simulink model "Chap7_OFDM"  (R2016a)
settings: Solver=VariableStepDiscrete  StartTime=0.0  StopTime=SimTime  RelTol=1e-3
InitFcn:
  | DopplerShift = 10; % 最大多普勒频移，单位Hz
  | % LTE EPA信道模型
  | Tau = ([0 30 70 90 110 190 410]) * 1e-9; % 每径的延迟，单位s
  | Pdb = [0 -1.0 -2.0 -3.0 -8.0 -17.2 -20.8]; % 每径的功率衰减
  | SNR = 10; % 信噪比
  | SimTime = 5; % 仿真时间
undefined symbols (not defined in the file or in its folder): clock
libraries: dspmtrx3 x12, dspxfrm3 x4, commchan3 x3, commdigbbndam3 x3, commrandsrc2 x2, commsink2 x1
settings Model: Creator=Administrator  LastModifiedBy=Administrator
settings DataIOCC: LimitDataPoints=on  SaveFormat=Array
settings DebuggingCC: SignalRangeChecking=warning  ParameterOverflowMsg=warning  ParameterPrecisionLossMsg=none  ParameterTunabilityLossMsg=none
settings HardwareCC: ProdBitPerPointer=32  ProdLargestAtomicFloat=None  ProdIntDivRoundTo=Undefined  ProdEndianess=Unspecified  ProdWordSize=32  ProdHWDeviceType=ASIC/FPGA->ASIC/FPGA  TargetHWDeviceType=Generic->Custom  ProdEqTarget=off
settings ModelReferenceCC: PropagateSignalLabelsOutOfModel=off
settings ConfigComp: CovModelRefEnable=Off

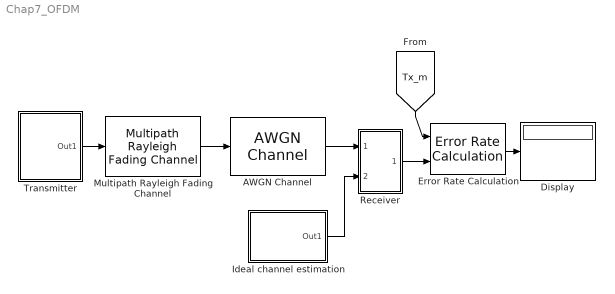
== system Chap7_OFDM ==
  AWGN Channel : commchan3/AWGN Channel  InputProcessing=Columns as channels (frame based)  seed=67  noiseMode=Variance from mask  EbNodB=10  EsNodB=10  SNRdB=10  bitsPerSym=1  Ps=1  Tsym=1  variance=1200/2048/(10^(SNR/10))
  Display : Display
  Error Rate Calculation : commsink2/Error Rate Calculation  N=0  st_delay=0  cp_mode=Entire frame  subframe=[]  PMode=Port  WsName=ErrorVec  RsMode2=off  stop=off  numErr=100  maxBits=1e6
  Ideal channel estimation : Subsystem
  Multipath Rayleigh Fading Channel : commchan3/Multipath Rayleigh Fading Channel  maxDopplerShift=10  spectrumType=Jakes  sigmaGaussian=1/sqrt(2)  coeffRounded=[1 -1.72 0.785]  freqMinMaxRJakes=[0 1]  freqMinMaxAJakes=[0 1]  sigmaGaussian1=1/sqrt(2)  sigmaGaussian2=1/sqrt(2)  centerFreqGaussian1=0.0  centerFreqGaussian2=0.0  gainGaussian1=0.5  gainGaussian2=0.5  coeffBell=9  dopplerSpectrum=doppler.jakes  pathDelays=Tau  avgPathGaindB=Pdb  normalizePathGains=on  seed=73  enableProbe=0  openVisAtStart=off  outPathGains=off  outDelay=off
  Receiver : Subsystem
  Transmitter : Subsystem
  wires:
  Multipath Rayleigh Fading Channel/1 -> AWGN Channel/1
  Error Rate Calculation/1 -> Display/1
  Transmitter/1(Out1) -> Multipath Rayleigh Fading Channel/1
  AWGN Channel/1 -> Receiver/1(In1)
  Ideal channel estimation/1(Out1) -> Receiver/2(In2)
  Receiver/1(Out1) -> Error Rate Calculation/2
  [Tx_m] -> Error Rate Calculation/1

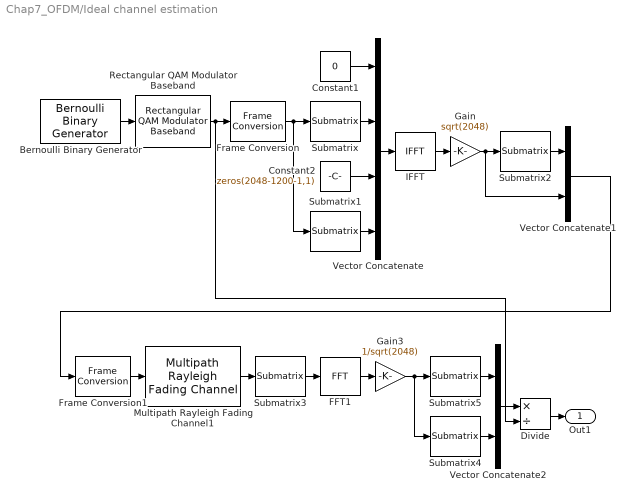
== system Chap7_OFDM/Ideal channel estimation ==
  Bernoulli Binary Generator : commrandsrc2/Bernoulli Binary Generator  P=0  seed=round(100*sum(clock))  Ts=0.5e-3/(1200*4)  frameBased=on  sampPerFrame=1200*4  orient=off  outDataType=double
  Constant1 : Constant  Value=0
  Constant2 : Constant  Value=zeros(2048-1200-1,1)
  Divide : Product  Inputs=*/
  FFT1 : dspxfrm3/FFT  FFTImplementation=Auto  CompMethod=Table lookup  TableOpt=NEW  TableOptActive=Speed  BitRevOrder=off  Normalize=off  InheritFFTLength=on  FFTLength=64  WrapInput=on  roundingMode=Floor  overflowMode=off  firstCoeffDataTypeStr=Inherit: Same word length as input  firstCoeffLastDataTypeStr=Inherit: Same word length as input  outputMin=[]  outputMax=[]
  Frame Conversion : FrameConversion  InheritSamplingMode=off  OutFrame=Sample-based
  Frame Conversion1 : FrameConversion  InheritSamplingMode=off
  Gain : Gain  Gain=sqrt(2048)
  Gain3 : Gain  Gain=1/sqrt(2048)
  IFFT : dspxfrm3/IFFT  FFTImplementation=Auto  CompMethod=Table lookup  TableOpt=NEW  TableOptActive=Speed  BitRevOrder=off  cs_in=off  Normalize=on  InheritFFTLength=on  FFTLength=64  WrapInput=on  mode=Complex  outSamplingMode=Sample based  roundingMode=Floor  overflowMode=off  firstCoeffDataTypeStr=Inherit: Same word length as input  firstCoeffLastDataTypeStr=Inherit: Same word length as input  outputMin=[]  outputMax=[]
  Multipath Rayleigh Fading Channel1 : commchan3/Multipath Rayleigh Fading Channel  maxDopplerShift=DopplerShift  spectrumType=Jakes  sigmaGaussian=1/sqrt(2)  coeffRounded=[1 -1.72 0.785]  freqMinMaxRJakes=[0 1]  freqMinMaxAJakes=[0 1]  sigmaGaussian1=1/sqrt(2)  sigmaGaussian2=1/sqrt(2)  centerFreqGaussian1=0.0  centerFreqGaussian2=0.0  gainGaussian1=0.5  gainGaussian2=0.5  coeffBell=9  dopplerSpectrum=doppler.jakes  pathDelays=Tau  avgPathGaindB=Pdb  normalizePathGains=on  seed=73  enableProbe=0  openVisAtStart=off  outPathGains=off  outDelay=off
  Rectangular QAM Modulator Baseband : commdigbbndam3/Rectangular QAM Modulator Baseband  M=16  InType=Bit  Enc=Gray  Mapping=[0:15]  PowType=Average Power  MinDist=2  AvgPow=1  PeakPow=1  Ph=0  outDtype=double  outWordLen=16  outUDDataType=sfix(16)  outFracLenMode=Best precision  outFracLen=15  outDataTypeStr=double  outLastDataTypeStr=double
  Submatrix : dspmtrx3/Submatrix  RowSpan=Range of rows  RowStartMode=Index  RowStartIndex=601  RowEndMode=Last  RowEndIndex=600  ColSpan=All columns  ColStartMode=First  ColStartIndex=1  ColEndMode=Last  ColEndIndex=1
  Submatrix1 : dspmtrx3/Submatrix  RowSpan=Range of rows  RowStartMode=First  RowStartIndex=1  RowEndMode=Index  RowEndIndex=600  ColSpan=All columns  ColStartMode=First  ColStartIndex=1  ColEndMode=Last  ColEndIndex=1
  Submatrix2 : dspmtrx3/Submatrix  RowSpan=Range of rows  RowStartMode=Index  RowStartIndex=2048-144+1  RowEndMode=Last  RowEndIndex=600  ColSpan=All columns  ColStartMode=First  ColStartIndex=1  ColEndMode=Last  ColEndIndex=1
  Submatrix3 : dspmtrx3/Submatrix  RowSpan=Range of rows  RowStartMode=Index  RowStartIndex=145  RowEndMode=Last  RowEndIndex=600  ColSpan=All columns  ColStartMode=First  ColStartIndex=1  ColEndMode=Last  ColEndIndex=1
  Submatrix4 : dspmtrx3/Submatrix  RowSpan=Range of rows  RowStartMode=Index  RowStartIndex=2  RowEndMode=Index  RowEndIndex=601  ColSpan=Range of columns  ColStartMode=First  ColStartIndex=1  ColEndMode=Last  ColEndIndex=1
  Submatrix5 : dspmtrx3/Submatrix  RowSpan=Range of rows  RowStartMode=Index  RowStartIndex=2048-600+1  RowEndMode=Last  RowEndIndex=600  ColSpan=Range of columns  ColStartMode=First  ColStartIndex=1  ColEndMode=Last  ColEndIndex=1
  Vector Concatenate : Concatenate  NumInputs=4
  Vector Concatenate1 : Concatenate
  Vector Concatenate2 : Concatenate
  Out1 : Outport
  wires:
  Frame Conversion/1 -> Submatrix1/1, Submatrix/1
  IFFT/1 -> Gain/1
  Submatrix/1 -> Vector Concatenate/2
  Constant1/1 -> Vector Concatenate/1
  Submatrix1/1 -> Vector Concatenate/4
  Constant2/1 -> Vector Concatenate/3
  Bernoulli Binary Generator/1 -> Rectangular QAM Modulator Baseband/1
  Vector Concatenate/1 -> IFFT/1
  Multipath Rayleigh Fading Channel1/1 -> Submatrix3/1
  FFT1/1 -> Gain3/1
  Submatrix5/1 -> Vector Concatenate2/1
  Submatrix4/1 -> Vector Concatenate2/2
  Vector Concatenate2/1 -> Divide/1
  Rectangular QAM Modulator Baseband/1 -> Divide/2, Frame Conversion/1
  Gain3/1 -> Submatrix5/1, Submatrix4/1
  Divide/1 -> Out1/1
  Gain/1 -> Vector Concatenate1/2, Submatrix2/1
  Submatrix2/1 -> Vector Concatenate1/1
  Vector Concatenate1/1 -> Frame Conversion1/1
  Frame Conversion1/1 -> Multipath Rayleigh Fading Channel1/1
  Submatrix3/1 -> FFT1/1

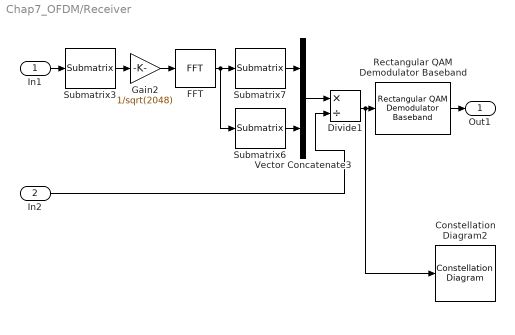
== system Chap7_OFDM/Receiver ==
  In1 : Inport
  In2 : Inport  Port=2
  Constellation Diagram2 : ConstellationDiagram
  Divide1 : Product  Inputs=*/
  FFT : dspxfrm3/FFT  FFTImplementation=Auto  CompMethod=Table lookup  TableOpt=NEW  TableOptActive=Speed  BitRevOrder=off  Normalize=off  InheritFFTLength=on  FFTLength=64  WrapInput=on  roundingMode=Floor  overflowMode=off  firstCoeffDataTypeStr=Inherit: Same word length as input  firstCoeffLastDataTypeStr=Inherit: Same word length as input  outputMin=[]  outputMax=[]
  Gain2 : Gain  Gain=1/sqrt(2048)
  Rectangular QAM Demodulator Baseband : commdigbbndam3/Rectangular QAM Demodulator Baseband  M=16  OutType=Bit  DecType=Hard decision  VarSource=Dialog  Variance=1  Dec=Gray  Mapping=[0:15]  PowType=Average Power  MinDist=2  AvgPow=1  PeakPow=1  Ph=0  outDtype1=Inherit via internal rule  outDtype2=Inherit via internal rule  derotateFactorWordLen=16  derotateFactorDataTypeStr=Inherit: Same word length as input  derotateFactorLastDataTypeStr=Inherit: Same word length as input  denormFactorWordLen=16  denormFactorDataTypeStr=Inherit: Same word length as input  denormFactorLastDataTypeStr=Inherit: Same word length as input  prodOutWordLen=32  prodOutOverflowMode=Wrap  prodOutRoundingMode=Floor  prodOutOvFlMode=off  prodOutOvFlModeLastStrValue=off  sumWordLen=32
  Submatrix3 : dspmtrx3/Submatrix  RowSpan=Range of rows  RowStartMode=Index  RowStartIndex=145  RowEndMode=Last  RowEndIndex=600  ColSpan=All columns  ColStartMode=First  ColStartIndex=1  ColEndMode=Last  ColEndIndex=1
  Submatrix6 : dspmtrx3/Submatrix  RowSpan=Range of rows  RowStartMode=Index  RowStartIndex=2  RowEndMode=Index  RowEndIndex=601  ColSpan=Range of columns  ColStartMode=First  ColStartIndex=1  ColEndMode=Last  ColEndIndex=1
  Submatrix7 : dspmtrx3/Submatrix  RowSpan=Range of rows  RowStartMode=Index  RowStartIndex=2048-600+1  RowEndMode=Last  RowEndIndex=600  ColSpan=Range of columns  ColStartMode=First  ColStartIndex=1  ColEndMode=Last  ColEndIndex=1
  Vector Concatenate3 : Concatenate
  Out1 : Outport
  wires:
  Rectangular QAM Demodulator Baseband/1 -> Out1/1
  In1/1 -> Submatrix3/1
  In2/1 -> Divide1/2
  Divide1/1 -> Constellation Diagram2/1, Rectangular QAM Demodulator Baseband/1
  Gain2/1 -> FFT/1
  Submatrix6/1 -> Vector Concatenate3/2
  Submatrix7/1 -> Vector Concatenate3/1
  FFT/1 -> Submatrix6/1, Submatrix7/1
  Vector Concatenate3/1 -> Divide1/1
  Submatrix3/1 -> Gain2/1

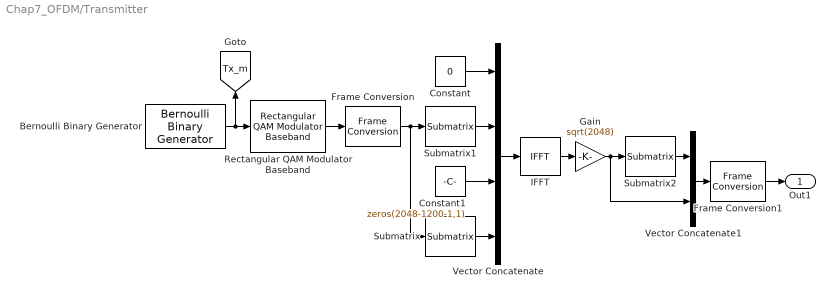
== system Chap7_OFDM/Transmitter ==
  Bernoulli Binary Generator : commrandsrc2/Bernoulli Binary Generator  P=0.5  seed=round(100*sum(clock))  Ts=0.5e-3/(1200*4)  frameBased=on  sampPerFrame=1200*4  orient=off  outDataType=double
  Constant : Constant  Value=0
  Constant1 : Constant  Value=zeros(2048-1200-1,1)
  Frame Conversion : FrameConversion  InheritSamplingMode=off  OutFrame=Sample-based
  Frame Conversion1 : FrameConversion  InheritSamplingMode=off
  Gain : Gain  Gain=sqrt(2048)
  IFFT : dspxfrm3/IFFT  FFTImplementation=Auto  CompMethod=Table lookup  TableOpt=NEW  TableOptActive=Speed  BitRevOrder=off  cs_in=off  Normalize=on  InheritFFTLength=on  FFTLength=64  WrapInput=on  mode=Complex  outSamplingMode=Sample based  roundingMode=Floor  overflowMode=off  firstCoeffDataTypeStr=Inherit: Same word length as input  firstCoeffLastDataTypeStr=Inherit: Same word length as input  outputMin=[]  outputMax=[]
  Rectangular QAM Modulator Baseband : commdigbbndam3/Rectangular QAM Modulator Baseband  M=16  InType=Bit  Enc=Gray  Mapping=[0:15]  PowType=Average Power  MinDist=2  AvgPow=1  PeakPow=1  Ph=0  outDtype=double  outWordLen=16  outUDDataType=sfix(16)  outFracLenMode=Best precision  outFracLen=15  outDataTypeStr=double  outLastDataTypeStr=double
  Submatrix : dspmtrx3/Submatrix  RowSpan=Range of rows  RowStartMode=First  RowStartIndex=1  RowEndMode=Index  RowEndIndex=600  ColSpan=All columns  ColStartMode=First  ColStartIndex=1  ColEndMode=Last  ColEndIndex=1
  Submatrix1 : dspmtrx3/Submatrix  RowSpan=Range of rows  RowStartMode=Index  RowStartIndex=601  RowEndMode=Last  RowEndIndex=600  ColSpan=All columns  ColStartMode=First  ColStartIndex=1  ColEndMode=Last  ColEndIndex=1
  Submatrix2 : dspmtrx3/Submatrix  RowSpan=Range of rows  RowStartMode=Index  RowStartIndex=2048-144+1  RowEndMode=Last  RowEndIndex=600  ColSpan=All columns  ColStartMode=First  ColStartIndex=1  ColEndMode=Last  ColEndIndex=1
  Vector Concatenate : Concatenate  NumInputs=4
  Vector Concatenate1 : Concatenate
  Out1 : Outport
  tag scope: Tx_m=global
  wires:
  Vector Concatenate/1 -> IFFT/1
  Bernoulli Binary Generator/1 -> [Tx_m], Rectangular QAM Modulator Baseband/1
  IFFT/1 -> Gain/1
  Constant1/1 -> Vector Concatenate/3
  Submatrix/1 -> Vector Concatenate/4
  Constant/1 -> Vector Concatenate/1
  Submatrix1/1 -> Vector Concatenate/2
  Rectangular QAM Modulator Baseband/1 -> Frame Conversion/1
  Frame Conversion/1 -> Submatrix1/1, Submatrix/1
  Gain/1 -> Vector Concatenate1/2, Submatrix2/1
  Submatrix2/1 -> Vector Concatenate1/1
  Vector Concatenate1/1 -> Frame Conversion1/1
  Frame Conversion1/1 -> Out1/1
